simulink model "t86"  (R2022b)
settings: Solver=VariableStepAuto  StartTime=0.0  StopTime=20  RelTol=1e-3
settings Model: Creator=mingh  LastModifiedBy=mingh

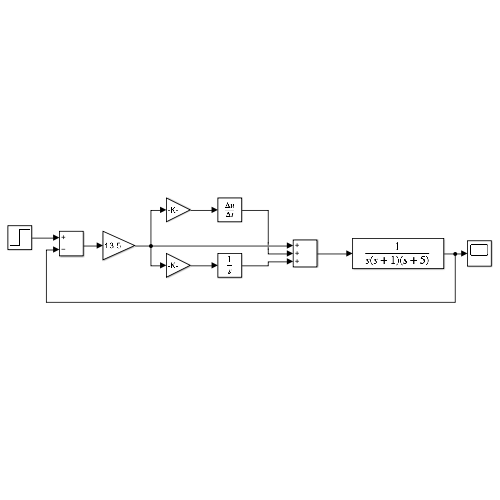
[thumbnail: Simulink's stored preview of the top-level diagram]
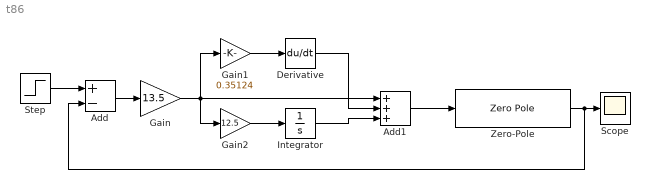
== system t86 ==
  Add : Sum  Inputs=+-
  Add1 : Sum  Inputs=+++
  Derivative : Derivative
  Gain : Gain  Gain=13.5
  Gain1 : Gain  Gain=0.35124
  Gain2 : Gain  Gain=12.5
  Integrator : Integrator
  Scope : Scope
  Step : Step  SampleTime=0
  Zero-Pole : ZeroPole  Zeros=[]  Poles=[0 -1 -5]  Gain=1
  wires:
  Step/1 -> Add/1
  Add/1 -> Gain/1
  Gain/1 -> Gain2/1, Add1/1, Gain1/1
  Gain1/1 -> Derivative/1
  Gain2/1 -> Integrator/1
  Add1/1 -> Zero-Pole/1
  Zero-Pole/1 -> Add/2, Scope/1
  Integrator/1 -> Add1/3
  Derivative/1 -> Add1/2
